simulink model "Ex3_3_sim"  (R2017b)
settings: Solver=ode45  StartTime=0.0  StopTime=0.2  RelTol=1e-3  EnableMultiTasking=on
undefined symbols (not defined in the file or in its folder): a0, a1, a2, b0
settings Model: Creator=Shin  LastModifiedBy=minakata
settings DataIOCC: LimitDataPoints=on  SaveFormat=Array
settings OptimizationCC: LifeSpan=inf
settings DebuggingCC: SolverPrmCheckMsg=warning  SFUnexpectedBacktrackingDiag=warning  SFNoUnconditionalDefaultTransitionDiag=warning  SFExecutionAtInitializationDiag=none
settings HardwareCC: ProdBitPerPointer=32  ProdBitPerSizeT=32  ProdBitPerPtrDiffT=32  ProdLargestAtomicFloat=None  ProdIntDivRoundTo=Undefined  ProdEndianess=Unspecified  ProdWordSize=32  ProdHWDeviceType=32-bit Generic
settings ModelReferenceCC: PropagateSignalLabelsOutOfModel=off
settings CodeAppCC: StateflowObjectComments=on
settings GRTTargetCC: TargetLangStandard=C89/C90 (ANSI)  GeneratePreprocessorConditionals=Disable all
settings ConfigComp: CovMetricSettings=dw  CovHtmlReporting=on  CovSaveCumulativeToWorkspaceVar=on  CovSaveSingleToWorkspaceVar=on  CovExternalEMLEnable=off  CovSFcnEnable=off

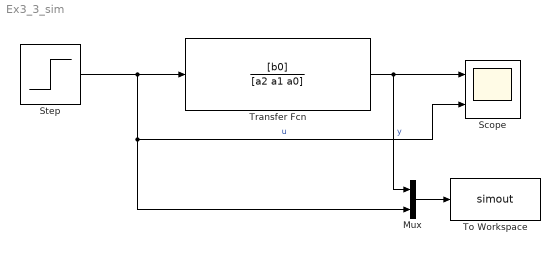
== system Ex3_3_sim ==
  Mux : Mux  Inputs=2
  Scope : Scope  NumInputPorts=2
  Step : Step  Time=0.01  SampleTime=0
  To Workspace : ToWorkspace  VariableName=simout  SaveFormat=Timeseries  SampleTime=-1
  Transfer Fcn : TransferFcn  Numerator=[b0]  Denominator=[a2 a1 a0]
  wires:
  Transfer Fcn/1 -> Mux/1, Scope/1  "y"
  Step/1 -> Transfer Fcn/1, Scope/2, Mux/2  "u"
  Mux/1 -> To Workspace/1
